simulink model "case6"  (R2024b)
settings: Solver=FixedStepAuto  StartTime=0  StopTime=1  FixedStep=1e-7  RelTol=1e-3
values from neighbouring files (symbols this model uses):
  SG_D_1_D = 0.01056    [IEEE9_case_parameters.m]    (also in case1_parameters.m; case2_parameters.m; case3_parameters.m; case4_parameters.m)
  SG_D_1_EnableSaturation = 0    [IEEE9_case_parameters.m]    (also in case1_parameters.m; case2_parameters.m; case3_parameters.m; case4_parameters.m)
  SG_D_1_f0 = 60    [IEEE9_case_parameters.m]    (also in case1_parameters.m; case2_parameters.m; case3_parameters.m; case4_parameters.m)
  SG_D_1_H = 7.5    [IEEE9_case_parameters.m]    (also in case1_parameters.m; case2_parameters.m; case3_parameters.m; case4_parameters.m)
  SG_D_1_K_A = 20    [IEEE9_case_parameters.m]    (also in case1_parameters.m; case2_parameters.m; case3_parameters.m; case4_parameters.m)
  SG_D_1_K_E = 1.000000e+1    (= 10)    [IEEE9_case_parameters.m]    (also in case1_parameters.m; case2_parameters.m; case3_parameters.m; case4_parameters.m)
  SG_D_1_K_F = 2.363    [IEEE9_case_parameters.m]    (also in case1_parameters.m; case2_parameters.m; case3_parameters.m; case4_parameters.m)
  SG_D_1_K_s = 0.5    [IEEE9_case_parameters.m]    (also in case1_parameters.m = 5; case2_parameters.m = 5; case3_parameters.m = 5; case4_parameters.m = 5)
  SG_D_1_R_a = 0.001088    [IEEE9_case_parameters.m]    (also in case1_parameters.m; case2_parameters.m; case3_parameters.m; case4_parameters.m)
  SG_D_1_S_A = 1    [IEEE9_case_parameters.m]    (also in case1_parameters.m; case2_parameters.m; case3_parameters.m; case4_parameters.m)
  SG_D_1_S_B = 0.103    [IEEE9_case_parameters.m]    (also in case1_parameters.m; case2_parameters.m; case3_parameters.m; case4_parameters.m)
  SG_D_1_S_N = 10.659857    [IEEE9_case_parameters.m]    (also in case1_parameters.m; case2_parameters.m; case3_parameters.m; case4_parameters.m)
  SG_D_1_SpeedPara = 200    [IEEE9_case_parameters.m]    (also in case1_parameters.m; case2_parameters.m; case3_parameters.m; case4_parameters.m)
  SG_D_1_T_0 = 0.720173    [IEEE9_case_parameters.m]    (also in case1_parameters.m = 0.755522; case2_parameters.m = 0.808931; case3_parameters.m = 0.869402; case4_parameters.m = 0.729316)
  SG_D_1_T_1 = 0.3    [IEEE9_case_parameters.m]    (also in case1_parameters.m; case2_parameters.m; case3_parameters.m; case4_parameters.m)
  SG_D_1_T_2 = 0.05    [IEEE9_case_parameters.m]    (also in case1_parameters.m; case2_parameters.m; case3_parameters.m; case4_parameters.m)
  SG_D_1_T_3 = 0.02    [IEEE9_case_parameters.m]    (also in case1_parameters.m; case2_parameters.m; case3_parameters.m; case4_parameters.m)
  SG_D_1_T_4 = 0.005    [IEEE9_case_parameters.m]    (also in case1_parameters.m; case2_parameters.m; case3_parameters.m; case4_parameters.m)
  SG_D_1_T_A = 0.02    [IEEE9_case_parameters.m]    (also in case1_parameters.m; case2_parameters.m; case3_parameters.m; case4_parameters.m)
  SG_D_1_T_dd = 8.000000e+0    (= 8)    [IEEE9_case_parameters.m]    (also in case1_parameters.m; case2_parameters.m; case3_parameters.m; case4_parameters.m)
  SG_D_1_T_ddd = 0.04    [IEEE9_case_parameters.m]    (also in case1_parameters.m; case2_parameters.m; case3_parameters.m; case4_parameters.m)
  SG_D_1_T_E = 0.314    [IEEE9_case_parameters.m]    (also in case1_parameters.m; case2_parameters.m; case3_parameters.m; case4_parameters.m)
  SG_D_1_T_F = 0.35    [IEEE9_case_parameters.m]    (also in case1_parameters.m; case2_parameters.m; case3_parameters.m; case4_parameters.m)
  SG_D_1_T_qd = 0.8    [IEEE9_case_parameters.m]    (also in case1_parameters.m; case2_parameters.m; case3_parameters.m; case4_parameters.m)
  SG_D_1_T_qdd = 0.02    [IEEE9_case_parameters.m]    (also in case1_parameters.m; case2_parameters.m; case3_parameters.m; case4_parameters.m)
  SG_D_1_T_speed = 0.1    [IEEE9_case_parameters.m]    (also in case1_parameters.m = 200; case2_parameters.m = 200; case3_parameters.m = 200; case4_parameters.m = 200)
  SG_D_1_T_w = 0.5    [IEEE9_case_parameters.m]    (also in case1_parameters.m; case2_parameters.m; case3_parameters.m; case4_parameters.m)
  SG_D_1_V_ref = 1.990276    [IEEE9_case_parameters.m]    (also in case1_parameters.m = 2.042296; case2_parameters.m = 2.051388; case3_parameters.m = 2.089584; case4_parameters.m = 2.01845)
  SG_D_1_w_ref = 376.991118    [IEEE9_case_parameters.m]    (also in case1_parameters.m; case2_parameters.m; case3_parameters.m; case4_parameters.m)
  SG_D_1_wb = 6.000000e+1    (= 60)    [IEEE9_case_parameters.m]    (also in case1_parameters.m; case2_parameters.m; case3_parameters.m; case4_parameters.m)
  SG_D_1_x_d = 1.9    [IEEE9_case_parameters.m]    (also in case1_parameters.m; case2_parameters.m; case3_parameters.m; case4_parameters.m)
  SG_D_1_x_dd = 0.302    [IEEE9_case_parameters.m]    (also in case1_parameters.m; case2_parameters.m; case3_parameters.m; case4_parameters.m)
  SG_D_1_x_ddd = 0.204    [IEEE9_case_parameters.m]    (also in case1_parameters.m; case2_parameters.m; case3_parameters.m; case4_parameters.m)
  SG_D_1_x_l = 0.05    [IEEE9_case_parameters.m]    (also in case1_parameters.m; case2_parameters.m; case3_parameters.m; case4_parameters.m)
  SG_D_1_x_q = 1.3    [IEEE9_case_parameters.m]    (also in case1_parameters.m; case2_parameters.m; case3_parameters.m; case4_parameters.m)
  SG_D_1_x_qd = 0.5    [IEEE9_case_parameters.m]    (also in case1_parameters.m; case2_parameters.m; case3_parameters.m; case4_parameters.m)
  SG_D_1_x_qdd = 0.3    [IEEE9_case_parameters.m]    (also in case1_parameters.m; case2_parameters.m; case3_parameters.m; case4_parameters.m)
  SG_D_2_D = 0.02    [IEEE9_case_parameters.m]    (also in case1_parameters.m; case2_parameters.m; case3_parameters.m; case4_parameters.m)
  SG_D_2_EnableSaturation = 0    [IEEE9_case_parameters.m]    (also in case1_parameters.m; case2_parameters.m; case3_parameters.m; case4_parameters.m)
  SG_D_2_f0 = 60    [IEEE9_case_parameters.m]    (also in case1_parameters.m; case2_parameters.m; case3_parameters.m; case4_parameters.m)
  SG_D_2_H = 8.000000e+0    (= 8)    [IEEE9_case_parameters.m]    (also in case1_parameters.m; case2_parameters.m; case3_parameters.m; case4_parameters.m)
  SG_D_2_K_A = 20    [IEEE9_case_parameters.m]    (also in case1_parameters.m; case2_parameters.m; case3_parameters.m; case4_parameters.m)
  SG_D_2_K_E = 1.000000e+1    (= 10)    [IEEE9_case_parameters.m]    (also in case1_parameters.m; case2_parameters.m; case3_parameters.m; case4_parameters.m)
  SG_D_2_K_F = 2.363    [IEEE9_case_parameters.m]    (also in case1_parameters.m; case2_parameters.m; case3_parameters.m; case4_parameters.m)
  SG_D_2_K_s = 0.5    [IEEE9_case_parameters.m]    (also in case1_parameters.m = 4; case2_parameters.m = 4; case3_parameters.m = 4; case4_parameters.m = 4)
  SG_D_2_R_a = 0.001088    [IEEE9_case_parameters.m]    (also in case1_parameters.m; case2_parameters.m; case3_parameters.m; case4_parameters.m)
  SG_D_2_S_A = 1    [IEEE9_case_parameters.m]    (also in case1_parameters.m; case2_parameters.m; case3_parameters.m; case4_parameters.m)
  SG_D_2_S_B = 0.103    [IEEE9_case_parameters.m]    (also in case1_parameters.m; case2_parameters.m; case3_parameters.m; case4_parameters.m)
  SG_D_2_S_N = 10.659857    [IEEE9_case_parameters.m]    (also in case1_parameters.m; case2_parameters.m; case3_parameters.m; case4_parameters.m)
  SG_D_2_SpeedPara = 200    [IEEE9_case_parameters.m]    (also in case1_parameters.m; case2_parameters.m; case3_parameters.m; case4_parameters.m)
  SG_D_2_T_0 = 1.632913    [IEEE9_case_parameters.m]    (also in case1_parameters.m = 1.632925; case2_parameters.m = 1.632915; case3_parameters.m = 1.632914; case4_parameters.m = 1.632927)
  SG_D_2_T_1 = 0.2    [IEEE9_case_parameters.m]    (also in case1_parameters.m; case2_parameters.m; case3_parameters.m; case4_parameters.m)
  SG_D_2_T_2 = 0.05    [IEEE9_case_parameters.m]    (also in case1_parameters.m; case2_parameters.m; case3_parameters.m; case4_parameters.m)
  SG_D_2_T_3 = 0.02    [IEEE9_case_parameters.m]    (also in case1_parameters.m; case2_parameters.m; case3_parameters.m; case4_parameters.m)
  SG_D_2_T_4 = 0.005    [IEEE9_case_parameters.m]    (also in case1_parameters.m; case2_parameters.m; case3_parameters.m; case4_parameters.m)
  SG_D_2_T_A = 0.02    [IEEE9_case_parameters.m]    (also in case1_parameters.m; case2_parameters.m; case3_parameters.m; case4_parameters.m)
  SG_D_2_T_dd = 7.9    [IEEE9_case_parameters.m]    (also in case1_parameters.m; case2_parameters.m; case3_parameters.m; case4_parameters.m)
  SG_D_2_T_ddd = 0.04    [IEEE9_case_parameters.m]    (also in case1_parameters.m; case2_parameters.m; case3_parameters.m; case4_parameters.m)
  SG_D_2_T_E = 0.314    [IEEE9_case_parameters.m]    (also in case1_parameters.m; case2_parameters.m; case3_parameters.m; case4_parameters.m)
  SG_D_2_T_F = 0.35    [IEEE9_case_parameters.m]    (also in case1_parameters.m; case2_parameters.m; case3_parameters.m; case4_parameters.m)
  SG_D_2_T_qd = 0.8    [IEEE9_case_parameters.m]    (also in case1_parameters.m; case2_parameters.m; case3_parameters.m; case4_parameters.m)
  SG_D_2_T_qdd = 0.015    [IEEE9_case_parameters.m]    (also in case1_parameters.m; case2_parameters.m; case3_parameters.m; case4_parameters.m)
  SG_D_2_T_speed = 0.1    [IEEE9_case_parameters.m]    (also in case1_parameters.m = 150; case2_parameters.m = 150; case3_parameters.m = 150; case4_parameters.m = 150)
  SG_D_2_T_w = 0.35    [IEEE9_case_parameters.m]    (also in case1_parameters.m; case2_parameters.m; case3_parameters.m; case4_parameters.m)
  SG_D_2_V_ref = 2.58547    [IEEE9_case_parameters.m]    (also in case1_parameters.m = 2.597896; case2_parameters.m = 2.587136; case3_parameters.m = 2.586042; case4_parameters.m = 2.599679)
  SG_D_2_w_ref = 376.991118    [IEEE9_case_parameters.m]    (also in case1_parameters.m; case2_parameters.m; case3_parameters.m; case4_parameters.m)
  SG_D_2_wb = 6.000000e+1    (= 60)    [IEEE9_case_parameters.m]    (also in case1_parameters.m; case2_parameters.m; case3_parameters.m; case4_parameters.m)
  SG_D_2_x_d = 1.8    [IEEE9_case_parameters.m]    (also in case1_parameters.m; case2_parameters.m; case3_parameters.m; case4_parameters.m)
  SG_D_2_x_dd = 0.302    [IEEE9_case_parameters.m]    (also in case1_parameters.m; case2_parameters.m; case3_parameters.m; case4_parameters.m)
  SG_D_2_x_ddd = 0.204    [IEEE9_case_parameters.m]    (also in case1_parameters.m; case2_parameters.m; case3_parameters.m; case4_parameters.m)
  SG_D_2_x_l = 0.05    [IEEE9_case_parameters.m]    (also in case1_parameters.m; case2_parameters.m; case3_parameters.m; case4_parameters.m)
  SG_D_2_x_q = 1.25    [IEEE9_case_parameters.m]    (also in case1_parameters.m; case2_parameters.m; case3_parameters.m; case4_parameters.m)
  SG_D_2_x_qd = 0.5    [IEEE9_case_parameters.m]    (also in case1_parameters.m; case2_parameters.m; case3_parameters.m; case4_parameters.m)
  SG_D_2_x_qdd = 0.3    [IEEE9_case_parameters.m]    (also in case1_parameters.m; case2_parameters.m; case3_parameters.m; case4_parameters.m)
  SG_D_3_D = 0.02    [IEEE9_case_parameters.m]    (also in case1_parameters.m; case2_parameters.m; case3_parameters.m; case4_parameters.m)
  SG_D_3_EnableSaturation = 0    [IEEE9_case_parameters.m]    (also in case1_parameters.m; case2_parameters.m; case3_parameters.m; case4_parameters.m)
  SG_D_3_f0 = 60    [IEEE9_case_parameters.m]    (also in case1_parameters.m; case2_parameters.m; case3_parameters.m; case4_parameters.m)
  SG_D_3_H = 7.7    [IEEE9_case_parameters.m]    (also in case1_parameters.m; case2_parameters.m; case3_parameters.m; case4_parameters.m)
  SG_D_3_K_A = 20    [IEEE9_case_parameters.m]    (also in case1_parameters.m; case2_parameters.m; case3_parameters.m; case4_parameters.m)
  SG_D_3_K_E = 1.000000e+1    (= 10)    [IEEE9_case_parameters.m]    (also in case1_parameters.m; case2_parameters.m; case3_parameters.m; case4_parameters.m)
  SG_D_3_K_F = 2.363    [IEEE9_case_parameters.m]    (also in case1_parameters.m; case2_parameters.m; case3_parameters.m; case4_parameters.m)
  SG_D_3_K_s = 0.2    [IEEE9_case_parameters.m]    (also in case1_parameters.m = 2; case2_parameters.m = 2; case3_parameters.m = 2; case4_parameters.m = 2)
  SG_D_3_R_a = 0.001088    [IEEE9_case_parameters.m]    (also in case1_parameters.m; case2_parameters.m; case3_parameters.m; case4_parameters.m)
  SG_D_3_S_A = 1    [IEEE9_case_parameters.m]    (also in case1_parameters.m; case2_parameters.m; case3_parameters.m; case4_parameters.m)
  SG_D_3_S_B = 0.103    [IEEE9_case_parameters.m]    (also in case1_parameters.m; case2_parameters.m; case3_parameters.m; case4_parameters.m)
  SG_D_3_S_N = 10.659857    [IEEE9_case_parameters.m]    (also in case1_parameters.m; case2_parameters.m; case3_parameters.m; case4_parameters.m)
  SG_D_3_SpeedPara = 200    [IEEE9_case_parameters.m]    (also in case1_parameters.m; case2_parameters.m; case3_parameters.m; case4_parameters.m)
  SG_D_3_T_0 = 0.850788    [IEEE9_case_parameters.m]    (also in case1_parameters.m = 0.850786; case2_parameters.m = 0.850787; case3_parameters.m; case4_parameters.m = 0.850786)
  SG_D_3_T_1 = 0.2    [IEEE9_case_parameters.m]    (also in case1_parameters.m; case2_parameters.m; case3_parameters.m; case4_parameters.m)
  SG_D_3_T_2 = 0.05    [IEEE9_case_parameters.m]    (also in case1_parameters.m; case2_parameters.m; case3_parameters.m; case4_parameters.m)
  SG_D_3_T_3 = 0.02    [IEEE9_case_parameters.m]    (also in case1_parameters.m; case2_parameters.m; case3_parameters.m; case4_parameters.m)
  SG_D_3_T_4 = 0.005    [IEEE9_case_parameters.m]    (also in case1_parameters.m; case2_parameters.m; case3_parameters.m; case4_parameters.m)
  SG_D_3_T_A = 0.02    [IEEE9_case_parameters.m]    (also in case1_parameters.m; case2_parameters.m; case3_parameters.m; case4_parameters.m)
  SG_D_3_T_dd = 8.1    [IEEE9_case_parameters.m]    (also in case1_parameters.m; case2_parameters.m; case3_parameters.m; case4_parameters.m)
  SG_D_3_T_ddd = 0.04    [IEEE9_case_parameters.m]    (also in case1_parameters.m; case2_parameters.m; case3_parameters.m; case4_parameters.m)
  SG_D_3_T_E = 0.314    [IEEE9_case_parameters.m]    (also in case1_parameters.m; case2_parameters.m; case3_parameters.m; case4_parameters.m)
  SG_D_3_T_F = 0.35    [IEEE9_case_parameters.m]    (also in case1_parameters.m; case2_parameters.m; case3_parameters.m; case4_parameters.m)
  SG_D_3_T_qd = 0.8    [IEEE9_case_parameters.m]    (also in case1_parameters.m; case2_parameters.m; case3_parameters.m; case4_parameters.m)
  SG_D_3_T_qdd = 0.015    [IEEE9_case_parameters.m]    (also in case1_parameters.m; case2_parameters.m; case3_parameters.m; case4_parameters.m)
  SG_D_3_T_speed = 0.1    [IEEE9_case_parameters.m]    (also in case1_parameters.m = 180; case2_parameters.m = 180; case3_parameters.m = 180; case4_parameters.m = 180)
  SG_D_3_T_w = 0.4    [IEEE9_case_parameters.m]    (also in case1_parameters.m; case2_parameters.m; case3_parameters.m; case4_parameters.m)
  SG_D_3_V_ref = 1.892727    [IEEE9_case_parameters.m]    (also in case1_parameters.m = 1.906439; case2_parameters.m = 1.895535; case3_parameters.m = 1.892105; case4_parameters.m = 1.906598)
  SG_D_3_w_ref = 376.991118    [IEEE9_case_parameters.m]    (also in case1_parameters.m; case2_parameters.m; case3_parameters.m; case4_parameters.m)
  SG_D_3_wb = 6.000000e+1    (= 60)    [IEEE9_case_parameters.m]    (also in case1_parameters.m; case2_parameters.m; case3_parameters.m; case4_parameters.m)
  SG_D_3_x_d = 1.85    [IEEE9_case_parameters.m]    (also in case1_parameters.m; case2_parameters.m; case3_parameters.m; case4_parameters.m)
  SG_D_3_x_dd = 0.302    [IEEE9_case_parameters.m]    (also in case1_parameters.m; case2_parameters.m; case3_parameters.m; case4_parameters.m)
  SG_D_3_x_ddd = 0.204    [IEEE9_case_parameters.m]    (also in case1_parameters.m; case2_parameters.m; case3_parameters.m; case4_parameters.m)
  SG_D_3_x_l = 0.05    [IEEE9_case_parameters.m]    (also in case1_parameters.m; case2_parameters.m; case3_parameters.m; case4_parameters.m)
  SG_D_3_x_q = 1.2    [IEEE9_case_parameters.m]    (also in case1_parameters.m; case2_parameters.m; case3_parameters.m; case4_parameters.m)
  SG_D_3_x_qd = 0.5    [IEEE9_case_parameters.m]    (also in case1_parameters.m; case2_parameters.m; case3_parameters.m; case4_parameters.m)
  SG_D_3_x_qdd = 0.3    [IEEE9_case_parameters.m]    (also in case1_parameters.m; case2_parameters.m; case3_parameters.m; case4_parameters.m)
(part 9 of 12)

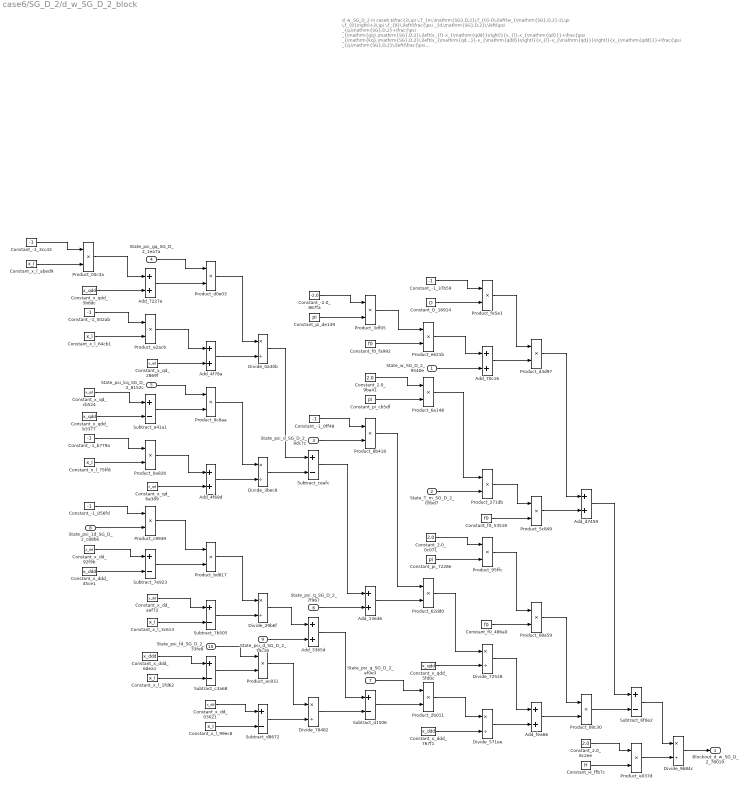
== system case6/SG_D_2/d_w_SG_D_2_block ==
  note: d_w_SG_D_2 in case6
      | $\frac{2\,\pi \,T_{m,\mathrm{SG},D,2}\,f_{0}-D\,\left(w_{\mathrm{SG},D,2}-2\,\pi \,f_{0}\right)+2\,\pi \,f_{0}\,\left(\frac{\psi _{d,\mathrm{SG},D,2}\,\left(\psi _{q,\mathrm{SG},D,2}+\frac{\psi _{\mathrm{gq},\mathrm{SG},D,2}\,\left(x_{l}-x_{\mathrm{qdd}}\right)}{x_{l}-x_{\mathrm{qd}}}+\frac{\psi _{\mathrm{kq},\mathrm{SG},D,2}\,\left(x_{\mathrm{qd}}-x_{\mathrm{qdd}}\right)}{x_{l}-x_{\mathrm{qd}}}\right)}{x_{\mathrm{qdd}}}+\frac{\psi _{q,\mathrm{SG},D,2}\,\left(\frac{\psi _{\mathrm{1d},\mathrm{SG},D,2}\,\left(x_{\mathrm{dd}}-x_{\mathrm{ddd}}\right)}{x_{\mathrm{dd}}-x_{l}}-\psi _{d,\mathrm{SG},D,2}+\frac{\psi _{\mathrm{fd},\mathrm{SG},D,2}\,\left(x_{\mathrm{ddd}}-x_{l}\right)}{x_{\mathrm{dd}}-x_{l}}\right)}{x_{\mathrm{ddd}}}\right)}{2\,H}$
      | Automatically generated on 2025-10-31 19:18:02 .
  State_w_SG_D_2_9540e : Inport
  State_T_m_SG_D_2_05bd7 : Inport  Port=2
  State_psi_d_SG_D_2_9dc7c : Inport  Port=3
  State_psi_gq_SG_D_2_1ea7a : Inport  Port=4
  State_psi_kq_SG_D_2_8152c : Inport  Port=5
  State_psi_q_SG_D_2_7f967 : Inport  Port=6
  State_psi_q_SG_D_2_af0e3 : Inport  Port=7
  State_psi_1d_SG_D_2_c88b6 : Inport  Port=8
  State_psi_d_SG_D_2_75c16 : Inport  Port=9
  State_psi_fd_SG_D_2_33fe8 : Inport  Port=10
  Add_13e46 : Sum
  Add_3365d : Sum
  Add_4f69d : Sum
  Add_4f78a : Sum
  Add_70c16 : Sum
  Add_7227e : Sum
  Add_d7459 : Sum
  Add_fea66 : Sum
  Constant_-1_056fd : Constant  Value=-1
  Constant_-1_0ff48 : Constant  Value=-1
  Constant_-1_37b59 : Constant  Value=-1
  Constant_-1_3cc43 : Constant  Value=-1
  Constant_-1_502ab : Constant  Value=-1
  Constant_-1_b779a : Constant  Value=-1
  Constant_-2.0_867fa : Constant  Value=-2.0
  Constant_2.0_0c071 : Constant  Value=2.0
  Constant_2.0_8c2ee : Constant  Value=2.0
  Constant_2.0_9ba41 : Constant  Value=2.0
  Constant_D_16914 : Constant  Value=D
  Constant_H_ffb7c : Constant  Value=H
  Constant_f0_486a0 : Constant  Value=f0
  Constant_f0_53518 : Constant  Value=f0
  Constant_f0_fa992 : Constant  Value=f0
  Constant_pi_7228e : Constant  Value=pi
  Constant_pi_cb5df : Constant  Value=pi
  Constant_pi_de149 : Constant  Value=pi
  Constant_x_dd_03021 : Constant  Value=x_dd
  Constant_x_dd_92f9b : Constant  Value=x_dd
  Constant_x_dd_aef72 : Constant  Value=x_dd
  Constant_x_ddd_45ce1 : Constant  Value=x_ddd
  Constant_x_ddd_6dea1 : Constant  Value=x_ddd
  Constant_x_ddd_767f1 : Constant  Value=x_ddd
  Constant_x_l_1fd62 : Constant  Value=x_l
  Constant_x_l_3c613 : Constant  Value=x_l
  Constant_x_l_64cb1 : Constant  Value=x_l
  Constant_x_l_75ff8 : Constant  Value=x_l
  Constant_x_l_99ec8 : Constant  Value=x_l
  Constant_x_l_abed9 : Constant  Value=x_l
  Constant_x_qd_2869f : Constant  Value=x_qd
  Constant_x_qd_6a389 : Constant  Value=x_qd
  Constant_x_qd_cb524 : Constant  Value=x_qd
  Constant_x_qdd_5b8dc : Constant  Value=x_qdd
  Constant_x_qdd_5fd0c : Constant  Value=x_qdd
  Constant_x_qdd_b3377 : Constant  Value=x_qdd
  Divide_0a30b : Product  Inputs=*/
  Divide_29b6f : Product  Inputs=*/
  Divide_3bec8 : Product  Inputs=*/
  Divide_571ee : Product  Inputs=*/
  Divide_72528 : Product  Inputs=*/
  Divide_78482 : Product  Inputs=*/
  Divide_9b84c : Product  Inputs=*/
  Product_05c3a : Product
  Product_08a59 : Product
  Product_08c30 : Product
  Product_0a826 : Product
  Product_271db : Product
  Product_2b011 : Product
  Product_3df05 : Product
  Product_5c849 : Product
  Product_62dd0 : Product
  Product_6a148 : Product
  Product_8b418 : Product
  Product_8c6aa : Product
  Product_95ffc : Product
  Product_ac831 : Product
  Product_bd817 : Product
  Product_c8949 : Product
  Product_d0e03 : Product
  Product_d3d97 : Product
  Product_e037d : Product
  Product_e2ac6 : Product
  Product_e621b : Product
  Product_fe5e1 : Product
  Subtract_6f0e2 : Sum  Inputs=+-
  Subtract_7b505 : Sum  Inputs=+-
  Subtract_7e923 : Sum  Inputs=+-
  Subtract_c3a68 : Sum  Inputs=+-
  Subtract_ceafc : Sum  Inputs=+-
  Subtract_d1506 : Sum  Inputs=+-
  Subtract_d8672 : Sum  Inputs=+-
  Subtract_e41a1 : Sum  Inputs=+-
  Blockout_d_w_SG_D_2_78019 : Outport
  wires:
  Constant_x_qd_cb524/1 -> Subtract_e41a1/1
  Constant_-1_b779a/1 -> Product_0a826/1
  Constant_-1_3cc43/1 -> Product_05c3a/1
  Constant_x_qdd_b3377/1 -> Subtract_e41a1/2
  Subtract_d8672/1 -> Divide_78482/2
  Constant_x_l_75ff8/1 -> Product_0a826/2
  Constant_x_l_abed9/1 -> Product_05c3a/2
  Product_0a826/1 -> Add_4f69d/1
  Product_05c3a/1 -> Add_7227e/1
  Constant_x_l_3c613/1 -> Subtract_7b505/2
  Constant_x_l_64cb1/1 -> Product_e2ac6/2
  Constant_x_ddd_767f1/1 -> Divide_571ee/2
  Subtract_c3a68/1 -> Product_ac831/2
  Constant_x_qd_6a389/1 -> Add_4f69d/2
  Constant_x_qdd_5b8dc/1 -> Add_7227e/2
  Constant_-1_502ab/1 -> Product_e2ac6/1
  State_psi_d_SG_D_2_9dc7c/1 -> Product_8b418/2
  Constant_-1_056fd/1 -> Product_c8949/1
  State_w_SG_D_2_9540e/1 -> Add_70c16/2
  Product_e2ac6/1 -> Add_4f78a/1
  State_psi_1d_SG_D_2_c88b6/1 -> Product_c8949/2
  Constant_x_dd_92f9b/1 -> Subtract_7e923/1
  Divide_0a30b/1 -> Subtract_ceafc/1
  Subtract_e41a1/1 -> Product_8c6aa/2
  Constant_x_ddd_45ce1/1 -> Subtract_7e923/2
  State_psi_gq_SG_D_2_1ea7a/1 -> Product_d0e03/1
  Add_4f69d/1 -> Divide_3bec8/2
  State_psi_d_SG_D_2_75c16/1 -> Add_3365d/2
  Add_7227e/1 -> Product_d0e03/2
  Constant_x_qd_2869f/1 -> Add_4f78a/2
  State_psi_kq_SG_D_2_8152c/1 -> Product_8c6aa/1
  Product_c8949/1 -> Product_bd817/1
  Subtract_7e923/1 -> Product_bd817/2
  Constant_pi_cb5df/1 -> Product_6a148/2
  Constant_x_dd_aef72/1 -> Subtract_7b505/1
  Constant_x_ddd_6dea1/1 -> Subtract_c3a68/1
  Constant_x_l_1fd62/1 -> Subtract_c3a68/2
  Product_d0e03/1 -> Divide_0a30b/1
  Add_4f78a/1 -> Divide_0a30b/2
  Add_13e46/1 -> Product_62dd0/2
  Product_8c6aa/1 -> Divide_3bec8/1
  Constant_pi_de149/1 -> Product_3df05/2
  Product_bd817/1 -> Divide_29b6f/1
  Subtract_7b505/1 -> Divide_29b6f/2
  State_psi_fd_SG_D_2_33fe8/1 -> Product_ac831/1
  Divide_29b6f/1 -> Add_3365d/1
  Constant_x_dd_03021/1 -> Subtract_d8672/1
  Constant_x_l_99ec8/1 -> Subtract_d8672/2
  Divide_3bec8/1 -> Subtract_ceafc/2
  Product_ac831/1 -> Divide_78482/1
  Constant_-1_0ff48/1 -> Product_8b418/1
  Constant_-2.0_867fa/1 -> Product_3df05/1
  Subtract_ceafc/1 -> Add_13e46/1
  Subtract_d1506/1 -> Product_2b011/2
  State_psi_q_SG_D_2_7f967/1 -> Add_13e46/2
  Constant_D_16914/1 -> Product_fe5e1/2
  Add_3365d/1 -> Subtract_d1506/1
  Divide_78482/1 -> Subtract_d1506/2
  Product_3df05/1 -> Product_e621b/1
  Constant_f0_fa992/1 -> Product_e621b/2
  Constant_2.0_9ba41/1 -> Product_6a148/1
  Product_8b418/1 -> Product_62dd0/1
  State_psi_q_SG_D_2_af0e3/1 -> Product_2b011/1
  Constant_-1_37b59/1 -> Product_fe5e1/1
  Product_e621b/1 -> Add_70c16/1
  Product_6a148/1 -> Product_271db/1
  State_T_m_SG_D_2_05bd7/1 -> Product_271db/2
  Constant_2.0_0c071/1 -> Product_95ffc/1
  Constant_pi_7228e/1 -> Product_95ffc/2
  Product_62dd0/1 -> Divide_72528/1
  Constant_x_qdd_5fd0c/1 -> Divide_72528/2
  Product_2b011/1 -> Divide_571ee/1
  Product_fe5e1/1 -> Product_d3d97/1
  Add_70c16/1 -> Product_d3d97/2
  Product_271db/1 -> Product_5c849/1
  Constant_f0_53518/1 -> Product_5c849/2
  Product_95ffc/1 -> Product_08a59/1
  Constant_f0_486a0/1 -> Product_08a59/2
  Divide_72528/1 -> Add_fea66/1
  Divide_571ee/1 -> Add_fea66/2
  Product_d3d97/1 -> Add_d7459/1
  Product_5c849/1 -> Add_d7459/2
  Product_08a59/1 -> Product_08c30/1
  Add_fea66/1 -> Product_08c30/2
  Add_d7459/1 -> Subtract_6f0e2/1
  Product_08c30/1 -> Subtract_6f0e2/2
  Constant_2.0_8c2ee/1 -> Product_e037d/1
  Constant_H_ffb7c/1 -> Product_e037d/2
  Subtract_6f0e2/1 -> Divide_9b84c/1
  Product_e037d/1 -> Divide_9b84c/2
  Divide_9b84c/1 -> Blockout_d_w_SG_D_2_78019/1

== system case6/SG_D_2/i_d_SG_D_2_block ==
  note: i_d_SG_D_2 in case6
      | $\frac{\sin\left(\theta _{\mathrm{SG},D,2}\right)\,\left(\frac{\psi _{\mathrm{1d},\mathrm{SG},D,2}\,\left(x_{\mathrm{dd}}-x_{\mathrm{ddd}}\right)}{x_{\mathrm{dd}}-x_{l}}-\psi _{d,\mathrm{SG},D,2}+\frac{\psi _{\mathrm{fd},\mathrm{SG},D,2}\,\left(x_{\mathrm{ddd}}-x_{l}\right)}{x_{\mathrm{dd}}-x_{l}}\right)}{x_{\mathrm{ddd}}}-\frac{\cos\left(\theta _{\mathrm{SG},D,2}\right)\,\left(\psi _{q,\mathrm{SG},D,2}+\frac{\psi _{\mathrm{gq},\mathrm{SG},D,2}\,\left(x_{l}-x_{\mathrm{qdd}}\right)}{x_{l}-x_{\mathrm{qd}}}+\frac{\psi _{\mathrm{kq},\mathrm{SG},D,2}\,\left(x_{\mathrm{qd}}-x_{\mathrm{qdd}}\right)}{x_{l}-x_{\mathrm{qd}}}\right)}{x_{\mathrm{qdd}}}$
      | Automatically generated on 2025-10-31 19:18:28 .
  State_psi_gq_SG_D_2_4eb5b : Inport
  State_psi_kq_SG_D_2_f39d8 : Inport  Port=2
  State_psi_q_SG_D_2_46eac : Inport  Port=3
  State_theta_SG_D_2_9c587 : Inport  Port=4
  State_psi_1d_SG_D_2_487b1 : Inport  Port=5
  State_psi_d_SG_D_2_503d3 : Inport  Port=6
  State_psi_fd_SG_D_2_72c98 : Inport  Port=7
  State_theta_SG_D_2_8a3e8 : Inport  Port=8
  Add_134e5 : Sum
  Add_47000 : Sum
  Add_73355 : Sum
  Add_e7760 : Sum
  Add_f4f94 : Sum
  Constant_-1_26789 : Constant  Value=-1
  Constant_-1_92fac : Constant  Value=-1
  Constant_-1_9aada : Constant  Value=-1
  Constant_-1_cc3f0 : Constant  Value=-1
  Constant_-1_d45b7 : Constant  Value=-1
  Constant_x_dd_0d9ed : Constant  Value=x_dd
  Constant_x_dd_a3116 : Constant  Value=x_dd
  Constant_x_dd_ac23f : Constant  Value=x_dd
  Constant_x_ddd_18541 : Constant  Value=x_ddd
  Constant_x_ddd_312a5 : Constant  Value=x_ddd
  Constant_x_ddd_da0d3 : Constant  Value=x_ddd
  Constant_x_l_30820 : Constant  Value=x_l
  Constant_x_l_aada1 : Constant  Value=x_l
  Constant_x_l_baaf7 : Constant  Value=x_l
  Constant_x_l_c4164 : Constant  Value=x_l
  Constant_x_l_e50dd : Constant  Value=x_l
  Constant_x_l_e8698 : Constant  Value=x_l
  Constant_x_qd_2efa0 : Constant  Value=x_qd
  Constant_x_qd_45eea : Constant  Value=x_qd
  Constant_x_qd_c6038 : Constant  Value=x_qd
  Constant_x_qdd_0ef5d : Constant  Value=x_qdd
  Constant_x_qdd_dead2 : Constant  Value=x_qdd
  Constant_x_qdd_e7ae0 : Constant  Value=x_qdd
  Divide_0e716 : Product  Inputs=*/
  Divide_33e19 : Product  Inputs=*/
  Divide_91359 : Product  Inputs=*/
  Divide_9cbd9 : Product  Inputs=*/
  Divide_c27e6 : Product  Inputs=*/
  Divide_cfa49 : Product  Inputs=*/
  MathFunc_cos_a6c8e : Trigonometry  Operator=cos
  MathFunc_sin_e7cf1 : Trigonometry
  Product_0e3ce : Product
  Product_125e9 : Product
  Product_1538c : Product
  Product_31ce8 : Product
  Product_47330 : Product
  Product_704c0 : Product
  Product_72a4c : Product
  Product_a2436 : Product
  Product_c5ad6 : Product
  Product_dda52 : Product
  Product_e5957 : Product
  Subtract_4ac4a : Sum  Inputs=+-
  Subtract_5108b : Sum  Inputs=+-
  Subtract_7d634 : Sum  Inputs=+-
  Subtract_7fb00 : Sum  Inputs=+-
  Subtract_9f5ae : Sum  Inputs=+-
  Subtract_ae266 : Sum  Inputs=+-
  Subtract_ae605 : Sum  Inputs=+-
  Subtract_cd3e2 : Sum  Inputs=+-
  Blockout_i_d_SG_D_2_1c8b0 : Outport
  wires:
  Constant_x_ddd_312a5/1 -> Subtract_4ac4a/1
  Constant_x_qd_c6038/1 -> Subtract_ae605/1
  Constant_-1_26789/1 -> Product_e5957/1
  Constant_-1_cc3f0/1 -> Product_1538c/1
  Subtract_7fb00/1 -> Blockout_i_d_SG_D_2_1c8b0/1
  Constant_x_qdd_e7ae0/1 -> Subtract_ae605/2
  Constant_x_l_e8698/1 -> Product_e5957/2
  Constant_x_l_aada1/1 -> Product_1538c/2
  Product_e5957/1 -> Add_f4f94/1
  Product_1538c/1 -> Add_134e5/1
  Constant_x_l_30820/1 -> Product_72a4c/2
  Constant_x_qd_45eea/1 -> Add_f4f94/2
  Constant_x_qdd_dead2/1 -> Add_134e5/2
  Constant_x_qdd_0ef5d/1 -> Divide_0e716/2
  MathFunc_cos_a6c8e/1 -> Product_704c0/2
  Constant_-1_d45b7/1 -> Product_72a4c/1
  State_psi_gq_SG_D_2_4eb5b/1 -> Product_c5ad6/1
  Subtract_4ac4a/1 -> Product_31ce8/2
  Product_dda52/1 -> Product_0e3ce/1
  Add_f4f94/1 -> Divide_33e19/2
  Add_134e5/1 -> Product_c5ad6/2
  Product_31ce8/1 -> Divide_91359/1
  Product_72a4c/1 -> Add_47000/1
  Constant_x_qd_2efa0/1 -> Add_47000/2
  State_theta_SG_D_2_8a3e8/1 -> MathFunc_sin_e7cf1/1
  State_psi_kq_SG_D_2_f39d8/1 -> Product_125e9/1
  Add_73355/1 -> Subtract_9f5ae/1
  Subtract_ae605/1 -> Product_125e9/2
  Product_c5ad6/1 -> Divide_cfa49/1
  Constant_-1_92fac/1 -> Product_dda52/1
  State_psi_1d_SG_D_2_487b1/1 -> Product_dda52/2
  State_psi_fd_SG_D_2_72c98/1 -> Product_31ce8/1
  Constant_x_dd_a3116/1 -> Subtract_5108b/1
  Product_0e3ce/1 -> Divide_c27e6/1
  Constant_x_ddd_18541/1 -> Subtract_5108b/2
  Divide_91359/1 -> Subtract_9f5ae/2
  Add_47000/1 -> Divide_cfa49/2
  Product_a2436/1 -> Divide_9cbd9/1
  Product_125e9/1 -> Divide_33e19/1
  Constant_-1_9aada/1 -> Product_47330/1
  Subtract_cd3e2/1 -> Divide_91359/2
  Subtract_5108b/1 -> Product_0e3ce/2
  Constant_x_dd_0d9ed/1 -> Subtract_ae266/1
  Subtract_9f5ae/1 -> Product_a2436/1
  Constant_x_l_e50dd/1 -> Subtract_ae266/2
  Constant_x_l_baaf7/1 -> Subtract_4ac4a/2
  Divide_cfa49/1 -> Subtract_7d634/1
  Divide_9cbd9/1 -> Subtract_7fb00/2
  Divide_33e19/1 -> Subtract_7d634/2
  Subtract_ae266/1 -> Divide_c27e6/2
  Constant_x_dd_ac23f/1 -> Subtract_cd3e2/1
  Divide_0e716/1 -> Subtract_7fb00/1
  Constant_x_l_c4164/1 -> Subtract_cd3e2/2
  Subtract_7d634/1 -> Add_e7760/1
  State_psi_q_SG_D_2_46eac/1 -> Add_e7760/2
  Constant_x_ddd_da0d3/1 -> Divide_9cbd9/2
  MathFunc_sin_e7cf1/1 -> Product_a2436/2
  Divide_c27e6/1 -> Add_73355/1
  State_psi_d_SG_D_2_503d3/1 -> Add_73355/2
  Add_e7760/1 -> Product_47330/2
  State_theta_SG_D_2_9c587/1 -> MathFunc_cos_a6c8e/1
  Product_47330/1 -> Product_704c0/1
  Product_704c0/1 -> Divide_0e716/1

== system case6/SG_D_2/i_q_SG_D_2_block ==
  note: i_q_SG_D_2 in case6
      | $-\frac{\sin\left(\theta _{\mathrm{SG},D,2}\right)\,\left(\psi _{q,\mathrm{SG},D,2}+\frac{\psi _{\mathrm{gq},\mathrm{SG},D,2}\,\left(x_{l}-x_{\mathrm{qdd}}\right)}{x_{l}-x_{\mathrm{qd}}}+\frac{\psi _{\mathrm{kq},\mathrm{SG},D,2}\,\left(x_{\mathrm{qd}}-x_{\mathrm{qdd}}\right)}{x_{l}-x_{\mathrm{qd}}}\right)}{x_{\mathrm{qdd}}}-\frac{\cos\left(\theta _{\mathrm{SG},D,2}\right)\,\left(\frac{\psi _{\mathrm{1d},\mathrm{SG},D,2}\,\left(x_{\mathrm{dd}}-x_{\mathrm{ddd}}\right)}{x_{\mathrm{dd}}-x_{l}}-\psi _{d,\mathrm{SG},D,2}+\frac{\psi _{\mathrm{fd},\mathrm{SG},D,2}\,\left(x_{\mathrm{ddd}}-x_{l}\right)}{x_{\mathrm{dd}}-x_{l}}\right)}{x_{\mathrm{ddd}}}$
      | Automatically generated on 2025-10-31 19:18:33 .
  State_psi_gq_SG_D_2_a612b : Inport
  State_psi_kq_SG_D_2_930b2 : Inport  Port=2
  State_psi_q_SG_D_2_e3c89 : Inport  Port=3
  State_theta_SG_D_2_df516 : Inport  Port=4
  State_psi_1d_SG_D_2_ac141 : Inport  Port=5
  State_psi_d_SG_D_2_f3333 : Inport  Port=6
  State_psi_fd_SG_D_2_0104a : Inport  Port=7
  State_theta_SG_D_2_4cc38 : Inport  Port=8
  Add_2cdc1 : Sum
  Add_36ef2 : Sum
  Add_5c10a : Sum
  Add_88abd : Sum
  Add_8c0f9 : Sum
  Add_d3d47 : Sum
  Constant_-1_2d138 : Constant  Value=-1
  Constant_-1_4cfb3 : Constant  Value=-1
  Constant_-1_8ad9f : Constant  Value=-1
  Constant_-1_99ea8 : Constant  Value=-1
  Constant_-1_c28d7 : Constant  Value=-1
  Constant_x_dd_29f39 : Constant  Value=x_dd
  Constant_x_dd_47f3e : Constant  Value=x_dd
  Constant_x_dd_b121b : Constant  Value=x_dd
  Constant_x_ddd_14015 : Constant  Value=x_ddd
  Constant_x_ddd_1a975 : Constant  Value=x_ddd
  Constant_x_ddd_4761c : Constant  Value=x_ddd
  Constant_x_l_039b6 : Constant  Value=x_l
  Constant_x_l_2bd38 : Constant  Value=x_l
  Constant_x_l_53d18 : Constant  Value=x_l
  Constant_x_l_65903 : Constant  Value=x_l
  Constant_x_l_d0455 : Constant  Value=x_l
  Constant_x_l_fb8ce : Constant  Value=x_l
  Constant_x_qd_997a8 : Constant  Value=x_qd
  Constant_x_qd_b7580 : Constant  Value=x_qd
  Constant_x_qd_e46e4 : Constant  Value=x_qd
  Constant_x_qdd_49a22 : Constant  Value=x_qdd
  Constant_x_qdd_74fe1 : Constant  Value=x_qdd
  Constant_x_qdd_f53f1 : Constant  Value=x_qdd
  Divide_36074 : Product  Inputs=*/
  Divide_56a4a : Product  Inputs=*/
  Divide_bc5de : Product  Inputs=*/
  Divide_d2f80 : Product  Inputs=*/
  Divide_d4cb0 : Product  Inputs=*/
  Divide_db70c : Product  Inputs=*/
  MathFunc_cos_e6aa8 : Trigonometry  Operator=cos
  MathFunc_sin_face3 : Trigonometry
  Product_0d390 : Product
  Product_1b9dd : Product
  Product_33b34 : Product
  Product_3eafc : Product
  Product_6937a : Product
  Product_82447 : Product
  Product_b7f8b : Product
  Product_cb2e8 : Product
  Product_eb929 : Product
  Product_f60e0 : Product
  Product_f6ad4 : Product
  Subtract_0681f : Sum  Inputs=+-
  Subtract_2a48f : Sum  Inputs=+-
  Subtract_5fa1c : Sum  Inputs=+-
  Subtract_68a2d : Sum  Inputs=+-
  Subtract_79f18 : Sum  Inputs=+-
  Subtract_86d0d : Sum  Inputs=+-
  Subtract_ef49e : Sum  Inputs=+-
  Blockout_i_q_SG_D_2_fe66f : Outport
  wires:
  MathFunc_sin_face3/1 -> Product_82447/2
  Product_3eafc/1 -> Product_82447/1
  Constant_-1_4cfb3/1 -> Product_0d390/1
  Constant_-1_99ea8/1 -> Product_f6ad4/1
  Constant_x_l_fb8ce/1 -> Product_0d390/2
  Product_0d390/1 -> Add_8c0f9/1
  Subtract_5fa1c/1 -> Product_cb2e8/2
  Constant_x_qdd_f53f1/1 -> Subtract_ef49e/2
  Constant_x_qdd_49a22/1 -> Add_8c0f9/2
  Add_5c10a/1 -> Product_3eafc/2
  Constant_x_l_2bd38/1 -> Product_f6ad4/2
  Constant_x_qd_b7580/1 -> Subtract_ef49e/1
  Constant_-1_8ad9f/1 -> Product_f60e0/1
  Constant_x_l_65903/1 -> Product_f60e0/2
  State_psi_1d_SG_D_2_ac141/1 -> Product_33b34/2
  State_psi_gq_SG_D_2_a612b/1 -> Product_b7f8b/1
  Add_8c0f9/1 -> Product_b7f8b/2
  Product_f6ad4/1 -> Add_36ef2/1
  Divide_db70c/1 -> Add_2cdc1/1
  Constant_x_qd_e46e4/1 -> Add_36ef2/2
  State_psi_kq_SG_D_2_930b2/1 -> Product_6937a/1
  Add_88abd/1 -> Subtract_0681f/1
  Constant_x_ddd_1a975/1 -> Subtract_5fa1c/2
  Subtract_ef49e/1 -> Product_6937a/2
  Product_f60e0/1 -> Add_d3d47/1
  Constant_x_qd_997a8/1 -> Add_d3d47/2
  Constant_-1_c28d7/1 -> Product_33b34/1
  Constant_x_l_d0455/1 -> Subtract_68a2d/2
  Constant_x_dd_47f3e/1 -> Subtract_5fa1c/1
  Product_b7f8b/1 -> Divide_bc5de/1
  Divide_36074/1 -> Subtract_0681f/2
  Add_36ef2/1 -> Divide_bc5de/2
  Product_eb929/1 -> Divide_d4cb0/1
  Product_6937a/1 -> Divide_d2f80/1
  Constant_-1_2d138/1 -> Product_3eafc/1
  Product_33b34/1 -> Product_cb2e8/1
  Add_d3d47/1 -> Divide_d2f80/2
  Constant_x_dd_b121b/1 -> Subtract_79f18/1
  Subtract_0681f/1 -> Product_eb929/1
  Subtract_2a48f/1 -> Product_1b9dd/2
  Constant_x_l_53d18/1 -> Subtract_79f18/2
  Constant_x_ddd_4761c/1 -> Subtract_2a48f/1
  Constant_x_l_039b6/1 -> Subtract_2a48f/2
  Divide_bc5de/1 -> Subtract_86d0d/1
  Divide_d4cb0/1 -> Add_2cdc1/2
  Product_1b9dd/1 -> Divide_36074/1
  Divide_d2f80/1 -> Subtract_86d0d/2
  Subtract_68a2d/1 -> Divide_36074/2
  Product_cb2e8/1 -> Divide_56a4a/1
  Subtract_79f18/1 -> Divide_56a4a/2
  Constant_x_qdd_74fe1/1 -> Divide_db70c/2
  State_psi_fd_SG_D_2_0104a/1 -> Product_1b9dd/1
  Constant_x_dd_29f39/1 -> Subtract_68a2d/1
  Subtract_86d0d/1 -> Add_5c10a/1
  State_psi_q_SG_D_2_e3c89/1 -> Add_5c10a/2
  Constant_x_ddd_14015/1 -> Divide_d4cb0/2
  Divide_56a4a/1 -> Add_88abd/1
  State_psi_d_SG_D_2_f3333/1 -> Add_88abd/2
  State_theta_SG_D_2_df516/1 -> MathFunc_sin_face3/1
  State_theta_SG_D_2_4cc38/1 -> MathFunc_cos_e6aa8/1
  MathFunc_cos_e6aa8/1 -> Product_eb929/2
  Product_82447/1 -> Divide_db70c/1
  Add_2cdc1/1 -> Blockout_i_q_SG_D_2_fe66f/1

== system case6/SG_D_2/theta_SG_D_2_out_block ==
  note: theta_SG_D_2_out in case6
      | $\theta _{\mathrm{SG},D,2}$
      | Automatically generated on 2025-10-31 19:18:39 .
  State_theta_SG_D_2_6ea16 : Inport
  Blockout_theta_SG_D_2_out_19715 : Outport
  wires:
  State_theta_SG_D_2_6ea16/1 -> Blockout_theta_SG_D_2_out_19715/1

== system case6/SG_D_2/w_SG_D_2_out_block ==
  note: w_SG_D_2_out in case6
      | $w_{\mathrm{SG},D,2}$
      | Automatically generated on 2025-10-31 19:18:39 .
  State_w_SG_D_2_a7da0 : Inport
  Blockout_w_SG_D_2_out_1bf45 : Outport
  wires:
  State_w_SG_D_2_a7da0/1 -> Blockout_w_SG_D_2_out_1bf45/1

== system case6/SG_D_3/T_e_SG_D_3_block ==
  note: T_e_SG_D_3 in case6
      | $-\frac{\psi _{d,\mathrm{SG},D,3}\,\left(\psi _{q,\mathrm{SG},D,3}+\frac{\psi _{\mathrm{gq},\mathrm{SG},D,3}\,\left(x_{l}-x_{\mathrm{qdd}}\right)}{x_{l}-x_{\mathrm{qd}}}+\frac{\psi _{\mathrm{kq},\mathrm{SG},D,3}\,\left(x_{\mathrm{qd}}-x_{\mathrm{qdd}}\right)}{x_{l}-x_{\mathrm{qd}}}\right)}{x_{\mathrm{qdd}}}-\frac{\psi _{q,\mathrm{SG},D,3}\,\left(\frac{\psi _{\mathrm{1d},\mathrm{SG},D,3}\,\left(x_{\mathrm{dd}}-x_{\mathrm{ddd}}\right)}{x_{\mathrm{dd}}-x_{l}}-\psi _{d,\mathrm{SG},D,3}+\frac{\psi _{\mathrm{fd},\mathrm{SG},D,3}\,\left(x_{\mathrm{ddd}}-x_{l}\right)}{x_{\mathrm{dd}}-x_{l}}\right)}{x_{\mathrm{ddd}}}$
      | Automatically generated on 2025-10-31 19:20:07 .
  State_psi_d_SG_D_3_8bdd5 : Inport
  State_psi_gq_SG_D_3_0552d : Inport  Port=2
  State_psi_kq_SG_D_3_0f4bf : Inport  Port=3
  State_psi_q_SG_D_3_17496 : Inport  Port=4
  State_psi_q_SG_D_3_1f719 : Inport  Port=5
  State_psi_1d_SG_D_3_b9c0b : Inport  Port=6
  State_psi_d_SG_D_3_c2826 : Inport  Port=7
  State_psi_fd_SG_D_3_9ec58 : Inport  Port=8
  Add_050fa : Sum
  Add_1ae52 : Sum
  Add_6fedf : Sum
  Add_749cb : Sum
  Add_a3764 : Sum
  Add_f207b : Sum
  Constant_-1_9bb5a : Constant  Value=-1
  Constant_-1_cb55a : Constant  Value=-1
  Constant_-1_cdc0c : Constant  Value=-1
  Constant_-1_d8286 : Constant  Value=-1
  Constant_-1_e010c : Constant  Value=-1
  Constant_x_dd_1a9fc : Constant  Value=x_dd
  Constant_x_dd_35836 : Constant  Value=x_dd
  Constant_x_dd_81f0e : Constant  Value=x_dd
  Constant_x_ddd_5f489 : Constant  Value=x_ddd
  Constant_x_ddd_78c38 : Constant  Value=x_ddd
  Constant_x_ddd_d691d : Constant  Value=x_ddd
  Constant_x_l_416b0 : Constant  Value=x_l
  Constant_x_l_4c493 : Constant  Value=x_l
  Constant_x_l_54ea5 : Constant  Value=x_l
  Constant_x_l_b6528 : Constant  Value=x_l
  Constant_x_l_c2def : Constant  Value=x_l
  Constant_x_l_d5f87 : Constant  Value=x_l
  Constant_x_qd_464b7 : Constant  Value=x_qd
  Constant_x_qd_9046a : Constant  Value=x_qd
  Constant_x_qd_cae54 : Constant  Value=x_qd
  Constant_x_qdd_5a360 : Constant  Value=x_qdd
  Constant_x_qdd_75dd7 : Constant  Value=x_qdd
  Constant_x_qdd_accc7 : Constant  Value=x_qdd
  Divide_02bb4 : Product  Inputs=*/
  Divide_2aade : Product  Inputs=*/
  Divide_8b0b1 : Product  Inputs=*/
  Divide_b2182 : Product  Inputs=*/
  Divide_cad6e : Product  Inputs=*/
  Divide_e5959 : Product  Inputs=*/
  Product_5f107 : Product
  Product_61e0a : Product
  Product_79b34 : Product
  Product_8e8b0 : Product
  Product_977d5 : Product
  Product_b3369 : Product
  Product_bfa4c : Product
  Product_c377d : Product
  Product_d976a : Product
  Product_de646 : Product
  Product_e7aec : Product
  Subtract_191cd : Sum  Inputs=+-
  Subtract_521c5 : Sum  Inputs=+-
  Subtract_73ae0 : Sum  Inputs=+-
  Subtract_db938 : Sum  Inputs=+-
  Subtract_e7cdf : Sum  Inputs=+-
  Subtract_f0f2a : Sum  Inputs=+-
  Subtract_fee3b : Sum  Inputs=+-
  Blockout_T_e_SG_D_3_697bf : Outport
  wires:
  State_psi_q_SG_D_3_17496/1 -> Add_749cb/2
  Constant_-1_cdc0c/1 -> Product_c377d/1
  Subtract_191cd/1 -> Product_79b34/2
  State_psi_1d_SG_D_3_b9c0b/1 -> Product_8e8b0/2
  Constant_-1_e010c/1 -> Product_61e0a/1
  Constant_x_l_416b0/1 -> Product_61e0a/2
  Add_050fa/1 -> Subtract_191cd/1
  State_psi_d_SG_D_3_c2826/1 -> Add_050fa/2
  Product_61e0a/1 -> Add_a3764/1
  Constant_x_qdd_75dd7/1 -> Subtract_73ae0/2
  Add_749cb/1 -> Product_de646/2
  Constant_x_qdd_accc7/1 -> Add_a3764/2
  State_psi_q_SG_D_3_1f719/1 -> Product_79b34/1
  Constant_x_l_b6528/1 -> Product_c377d/2
  Subtract_521c5/1 -> Divide_e5959/2
  Constant_x_l_c2def/1 -> Subtract_fee3b/2
  Constant_x_qd_464b7/1 -> Subtract_73ae0/1
  Constant_-1_cb55a/1 -> Product_977d5/1
  Subtract_f0f2a/1 -> Divide_b2182/2
  Constant_x_l_54ea5/1 -> Product_977d5/2
  Product_d976a/1 -> Divide_b2182/1
  Constant_-1_d8286/1 -> Product_8e8b0/1
  Product_8e8b0/1 -> Product_d976a/1
  Constant_x_dd_1a9fc/1 -> Subtract_e7cdf/1
  Constant_x_ddd_5f489/1 -> Subtract_e7cdf/2
  Add_6fedf/1 -> Blockout_T_e_SG_D_3_697bf/1
  State_psi_gq_SG_D_3_0552d/1 -> Product_5f107/1
  Product_79b34/1 -> Divide_02bb4/1
  Add_a3764/1 -> Product_5f107/2
  State_psi_fd_SG_D_3_9ec58/1 -> Product_bfa4c/1
  Product_c377d/1 -> Add_1ae52/1
  Constant_x_qd_cae54/1 -> Add_1ae52/2
  Constant_x_dd_35836/1 -> Subtract_f0f2a/1
  State_psi_kq_SG_D_3_0f4bf/1 -> Product_b3369/1
  Constant_x_dd_81f0e/1 -> Subtract_521c5/1
  Subtract_73ae0/1 -> Product_b3369/2
  Product_de646/1 -> Divide_2aade/1
  Product_977d5/1 -> Add_f207b/1
  Add_1ae52/1 -> Divide_8b0b1/2
  Constant_x_qd_9046a/1 -> Add_f207b/2
  Subtract_e7cdf/1 -> Product_d976a/2
  Constant_x_l_d5f87/1 -> Subtract_f0f2a/2
  Constant_x_ddd_78c38/1 -> Subtract_fee3b/1
  Product_5f107/1 -> Divide_8b0b1/1
  Product_b3369/1 -> Divide_cad6e/1
  Add_f207b/1 -> Divide_cad6e/2
  Constant_x_ddd_d691d/1 -> Divide_02bb4/2
  Subtract_fee3b/1 -> Product_bfa4c/2
  Divide_8b0b1/1 -> Subtract_db938/1
  Constant_x_l_4c493/1 -> Subtract_521c5/2
  Divide_cad6e/1 -> Subtract_db938/2
  Divide_b2182/1 -> Add_050fa/1
  Product_bfa4c/1 -> Divide_e5959/1
  Constant_-1_9bb5a/1 -> Product_e7aec/1
  State_psi_d_SG_D_3_8bdd5/1 -> Product_e7aec/2
  Subtract_db938/1 -> Add_749cb/1
  Divide_e5959/1 -> Subtract_191cd/2
  Product_e7aec/1 -> Product_de646/1
  Constant_x_qdd_5a360/1 -> Divide_2aade/2
  Divide_2aade/1 -> Add_6fedf/1
  Divide_02bb4/1 -> Add_6fedf/2

== system case6/SG_D_3/d_E_fd_SG_D_3_block ==
  note: d_E_fd_SG_D_3 in case6
      | $\frac{V_{f,\mathrm{SG},D,3}-E_{\mathrm{fd},\mathrm{SG},D,3}\,K_{E}}{T_{E}}$
      | Automatically generated on 2025-10-31 19:19:45 .
  State_E_fd_SG_D_3_b4832 : Inport
  State_V_f_SG_D_3_e8ba7 : Inport  Port=2
  Add_5f40e : Sum
  Constant_-1_d9e80 : Constant  Value=-1
  Constant_K_E_cd00a : Constant  Value=K_E
  Constant_T_E_2c390 : Constant  Value=T_E
  Divide_017b3 : Product  Inputs=*/
  Product_5c762 : Product
  Product_fd4af : Product
  Blockout_d_E_fd_SG_D_3_557e1 : Outport
  wires:
  State_V_f_SG_D_3_e8ba7/1 -> Add_5f40e/2
  Constant_-1_d9e80/1 -> Product_5c762/1
  State_E_fd_SG_D_3_b4832/1 -> Product_5c762/2
  Constant_T_E_2c390/1 -> Divide_017b3/2
  Product_5c762/1 -> Product_fd4af/1
  Product_fd4af/1 -> Add_5f40e/1
  Constant_K_E_cd00a/1 -> Product_fd4af/2
  Divide_017b3/1 -> Blockout_d_E_fd_SG_D_3_557e1/1
  Add_5f40e/1 -> Divide_017b3/1

== system case6/SG_D_3/d_Px_1_SG_D_3_block ==
  note: d_Px_1_SG_D_3 in case6
      | $\frac{w_{\mathrm{SG},D,3}-2\,\pi \,f_{0}}{T_{w}}-\frac{\mathrm{Px}_{1,\mathrm{SG},D,3}}{T_{w}}$
      | Automatically generated on 2025-10-31 19:19:46 .
  State_Px_1_SG_D_3_e4615 : Inport
  State_w_SG_D_3_9d504 : Inport  Port=2
  Add_8b31b : Sum
  Add_99a78 : Sum
  Constant_-1_63bba : Constant  Value=-1
  Constant_-2.0_4b2d7 : Constant  Value=-2.0
  Constant_T_w_819a0 : Constant  Value=T_w
  Constant_T_w_c0d79 : Constant  Value=T_w
  Constant_f0_79676 : Constant  Value=f0
  Constant_pi_8718a : Constant  Value=pi
  Divide_499e5 : Product  Inputs=*/
  Divide_c8771 : Product  Inputs=*/
  Product_22c9f : Product
  Product_549fb : Product
  Product_de403 : Product
  Blockout_d_Px_1_SG_D_3_53c6c : Outport
  wires:
  Constant_f0_79676/1 -> Product_de403/2
  Constant_-1_63bba/1 -> Product_549fb/1
  Constant_-2.0_4b2d7/1 -> Product_22c9f/1
  Constant_pi_8718a/1 -> Product_22c9f/2
  Product_22c9f/1 -> Product_de403/1
  State_w_SG_D_3_9d504/1 -> Add_99a78/2
  Divide_499e5/1 -> Add_8b31b/1
  State_Px_1_SG_D_3_e4615/1 -> Product_549fb/2
  Product_de403/1 -> Add_99a78/1
  Product_549fb/1 -> Divide_499e5/1
  Constant_T_w_c0d79/1 -> Divide_499e5/2
  Add_99a78/1 -> Divide_c8771/1
  Constant_T_w_819a0/1 -> Divide_c8771/2
  Divide_c8771/1 -> Add_8b31b/2
  Add_8b31b/1 -> Blockout_d_Px_1_SG_D_3_53c6c/1

== system case6/SG_D_3/d_Px_2_SG_D_3_block ==
  note: d_Px_2_SG_D_3 in case6
      | $\frac{\mathrm{Px}_{1,\mathrm{SG},D,3}-T_{2}\,\left(\frac{\mathrm{Px}_{1,\mathrm{SG},D,3}}{T_{w}}-\frac{w_{\mathrm{SG},D,3}-2\,\pi \,f_{0}}{T_{w}}\right)}{T_{1}}-\frac{\mathrm{Px}_{2,\mathrm{SG},D,3}}{T_{1}}$
      | Automatically generated on 2025-10-31 19:19:49 .
  State_Px_2_SG_D_3_c51e0 : Inport
  State_Px_1_SG_D_3_3f3ed : Inport  Port=2
  State_Px_1_SG_D_3_990a4 : Inport  Port=3
  State_w_SG_D_3_d4530 : Inport  Port=4
  Add_14230 : Sum
  Add_4519e : Sum
  Add_496c0 : Sum
  Add_bb12f : Sum
  Constant_-1_7c211 : Constant  Value=-1
  Constant_-1_f5ec4 : Constant  Value=-1
  Constant_-2.0_7ef49 : Constant  Value=-2.0
  Constant_T_1_67514 : Constant  Value=T_1
  Constant_T_1_b587f : Constant  Value=T_1
  Constant_T_2_0900e : Constant  Value=T_2
  Constant_T_w_3861c : Constant  Value=T_w
  Constant_T_w_f602f : Constant  Value=T_w
  Constant_f0_f7ac1 : Constant  Value=f0
  Constant_pi_f5d80 : Constant  Value=pi
  Divide_02d79 : Product  Inputs=*/
  Divide_0c98a : Product  Inputs=*/
  Divide_8f0d8 : Product  Inputs=*/
  Divide_b7b00 : Product  Inputs=*/
  Product_22067 : Product
  Product_31bd2 : Product
  Product_4358a : Product
  Product_df016 : Product
  Product_e9c0f : Product
  Blockout_d_Px_2_SG_D_3_5e411 : Outport
  wires:
  State_Px_1_SG_D_3_990a4/1 -> Product_df016/2
  Constant_-2.0_7ef49/1 -> Product_e9c0f/1
  Constant_f0_f7ac1/1 -> Product_22067/2
  Constant_pi_f5d80/1 -> Product_e9c0f/2
  Product_e9c0f/1 -> Product_22067/1
  State_w_SG_D_3_d4530/1 -> Add_bb12f/2
  Constant_-1_7c211/1 -> Product_df016/1
  Product_22067/1 -> Add_bb12f/1
  Product_df016/1 -> Divide_0c98a/1
  Constant_T_w_f602f/1 -> Divide_0c98a/2
  Add_bb12f/1 -> Divide_02d79/1
  Constant_T_w_3861c/1 -> Divide_02d79/2
  Divide_0c98a/1 -> Add_4519e/1
  Divide_02d79/1 -> Add_4519e/2
  Constant_T_2_0900e/1 -> Product_31bd2/1
  Add_4519e/1 -> Product_31bd2/2
  Constant_-1_f5ec4/1 -> Product_4358a/1
  Product_31bd2/1 -> Add_496c0/2
  State_Px_2_SG_D_3_c51e0/1 -> Product_4358a/2
  State_Px_1_SG_D_3_3f3ed/1 -> Add_496c0/1
  Product_4358a/1 -> Divide_b7b00/1
  Add_14230/1 -> Blockout_d_Px_2_SG_D_3_5e411/1
  Constant_T_1_b587f/1 -> Divide_b7b00/2
  Add_496c0/1 -> Divide_8f0d8/1
  Constant_T_1_67514/1 -> Divide_8f0d8/2
  Divide_b7b00/1 -> Add_14230/1
  Divide_8f0d8/1 -> Add_14230/2

== system case6/SG_D_3/d_Px_3_SG_D_3_block ==
  note: d_Px_3_SG_D_3 in case6
      | $\frac{\mathrm{Px}_{2,\mathrm{SG},D,3}+T_{4}\,\left(\frac{\mathrm{Px}_{1,\mathrm{SG},D,3}-T_{2}\,\left(\frac{\mathrm{Px}_{1,\mathrm{SG},D,3}}{T_{w}}-\frac{w_{\mathrm{SG},D,3}-2\,\pi \,f_{0}}{T_{w}}\right)}{T_{1}}-\frac{\mathrm{Px}_{2,\mathrm{SG},D,3}}{T_{1}}\right)}{T_{3}}-\frac{\mathrm{Px}_{3,\mathrm{SG},D,3}}{T_{3}}$
      | Automatically generated on 2025-10-31 19:19:52 .
  State_Px_3_SG_D_3_009d1 : Inport
  State_Px_2_SG_D_3_9ab37 : Inport  Port=2
  State_Px_2_SG_D_3_8a812 : Inport  Port=3
  State_Px_1_SG_D_3_51d69 : Inport  Port=4
  State_Px_1_SG_D_3_84b56 : Inport  Port=5
  State_w_SG_D_3_25f91 : Inport  Port=6
  Add_5c277 : Sum
  Add_6a657 : Sum
  Add_8c31f : Sum
  Add_9e8b1 : Sum
  Add_a6d1b : Sum
  Add_ecd23 : Sum
  Constant_-1_90b68 : Constant  Value=-1
  Constant_-1_98d9f : Constant  Value=-1
  Constant_-1_d7bba : Constant  Value=-1
  Constant_-2.0_41c0c : Constant  Value=-2.0
  Constant_T_1_27c18 : Constant  Value=T_1
  Constant_T_1_7a632 : Constant  Value=T_1
  Constant_T_2_39456 : Constant  Value=T_2
  Constant_T_3_417f1 : Constant  Value=T_3
  Constant_T_3_5e651 : Constant  Value=T_3
  Constant_T_4_8a82b : Constant  Value=T_4
  Constant_T_w_4f9dd : Constant  Value=T_w
  Constant_T_w_eb751 : Constant  Value=T_w
  Constant_f0_95211 : Constant  Value=f0
  Constant_pi_85041 : Constant  Value=pi
  Divide_0c590 : Product  Inputs=*/
  Divide_37421 : Product  Inputs=*/
  Divide_90a4b : Product  Inputs=*/
  Divide_9252b : Product  Inputs=*/
  Divide_c514a : Product  Inputs=*/
  Divide_e7914 : Product  Inputs=*/
  Product_1df6f : Product
  Product_24dba : Product
  Product_32013 : Product
  Product_755bb : Product
  Product_88102 : Product
  Product_ba320 : Product
  Product_e3291 : Product
  Blockout_d_Px_3_SG_D_3_ed081 : Outport
  wires:
  State_Px_1_SG_D_3_84b56/1 -> Product_e3291/2
  Constant_f0_95211/1 -> Product_24dba/2
  Constant_-2.0_41c0c/1 -> Product_1df6f/1
  Add_5c277/1 -> Divide_90a4b/1
  Constant_pi_85041/1 -> Product_1df6f/2
  Product_1df6f/1 -> Product_24dba/1
  State_w_SG_D_3_25f91/1 -> Add_6a657/2
  Constant_T_w_eb751/1 -> Divide_37421/2
  Constant_-1_98d9f/1 -> Product_e3291/1
  Product_24dba/1 -> Add_6a657/1
  Product_e3291/1 -> Divide_37421/1
  Add_6a657/1 -> Divide_9252b/1
  Product_755bb/1 -> Divide_c514a/1
  Constant_T_w_4f9dd/1 -> Divide_9252b/2
  Divide_37421/1 -> Add_a6d1b/1
  Divide_9252b/1 -> Add_a6d1b/2
  Constant_T_2_39456/1 -> Product_ba320/1
  Add_a6d1b/1 -> Product_ba320/2
  Constant_-1_d7bba/1 -> Product_755bb/1
  State_Px_2_SG_D_3_8a812/1 -> Product_755bb/2
  State_Px_1_SG_D_3_51d69/1 -> Add_5c277/1
  Constant_T_3_5e651/1 -> Divide_0c590/2
  Product_ba320/1 -> Add_5c277/2
  Constant_T_1_27c18/1 -> Divide_c514a/2
  Add_ecd23/1 -> Product_32013/2
  Constant_T_1_7a632/1 -> Divide_90a4b/2
  Divide_e7914/1 -> Add_9e8b1/2
  Divide_c514a/1 -> Add_ecd23/1
  Divide_90a4b/1 -> Add_ecd23/2
  Constant_T_4_8a82b/1 -> Product_32013/1
  Constant_-1_90b68/1 -> Product_88102/1
  State_Px_3_SG_D_3_009d1/1 -> Product_88102/2
  State_Px_2_SG_D_3_9ab37/1 -> Add_8c31f/1
  Product_32013/1 -> Add_8c31f/2
  Product_88102/1 -> Divide_0c590/1
  Add_8c31f/1 -> Divide_e7914/1
  Constant_T_3_417f1/1 -> Divide_e7914/2
  Divide_0c590/1 -> Add_9e8b1/1
  Add_9e8b1/1 -> Blockout_d_Px_3_SG_D_3_ed081/1
